simulink model "gm_NCO_32"  (R2023b)
settings: Solver=VariableStepAuto  StartTime=0.0  StopTime=100  RelTol=1e-3
undefined symbols (not defined in the file or in its folder): bhi
libraries: dsphdlfiltering2 x1, dsphdlsigops2 x1
settings Model: Creator=31651  LastModifiedBy=31651
settings OptimizationCC: BlockReduction=off  ConditionallyExecuteInputs=off  DefaultParameterBehavior=Inlined
settings DebuggingCC: AlgebraicLoopMsg=error  InheritedTsInSrcMsg=none
settings HardwareCC: ProdBitPerPointer=32  ProdBitPerSizeT=32  ProdBitPerPtrDiffT=32  ProdLargestAtomicFloat=None  ProdIntDivRoundTo=Undefined  ProdEndianess=Unspecified  ProdWordSize=32  ProdHWDeviceType=ASIC/FPGA->ASIC/FPGA  TargetBitPerPointer=64  TargetBitPerSizeT=64  TargetBitPerPtrDiffT=64  TargetLongLongMode=on  TargetIntDivRoundTo=Zero  TargetEndianess=LittleEndian  TargetWordSize=64  TargetHWDeviceType=Custom Processor->MATLAB Host Computer  ProdEqTarget=off

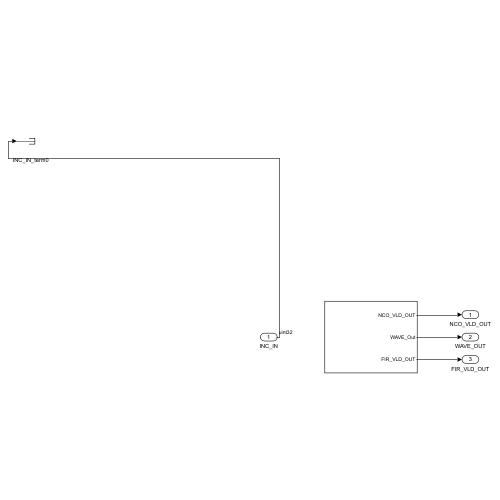
[thumbnail: Simulink's stored preview of the top-level diagram]
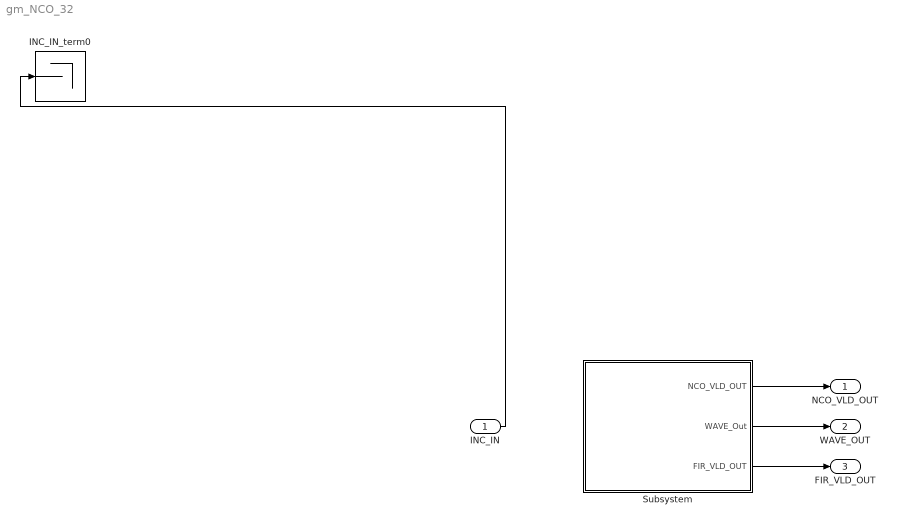
== system gm_NCO_32 ==
  INC_IN : Inport  OutDataTypeStr=uint32  PortDimensions=1  SampleTime=0.001
  INC_IN_term0 : Terminator
  Subsystem : Subsystem
  NCO_VLD_OUT : Outport  SampleTime=0.001  VectorParamsAs1DForOutWhenUnconnected=off
  WAVE_OUT : Outport  Port=2  SampleTime=0.001  VectorParamsAs1DForOutWhenUnconnected=off
  FIR_VLD_OUT : Outport  Port=3  SampleTime=0.001  VectorParamsAs1DForOutWhenUnconnected=off
  wires:
  INC_IN/1 -> INC_IN_term0/1
  Subsystem/1(NCO_VLD_OUT) -> NCO_VLD_OUT/1
  Subsystem/2(WAVE_Out) -> WAVE_OUT/1
  Subsystem/3(FIR_VLD_OUT) -> FIR_VLD_OUT/1

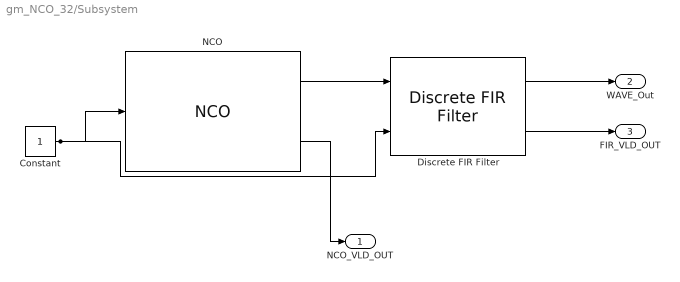
== system gm_NCO_32/Subsystem ==
  Constant : Constant  OutDataTypeStr=boolean  SampleTime=0.001
  Discrete FIR Filter : dsphdlfiltering2/Discrete FIR Filter  NumeratorSource=Property  Numerator=bhi  NumeratorPrototype=[]  FilterStructure=Direct form systolic  SerializationOption=Minimum number of cycles between valid input samples  NumCycles=2  NumberOfMultipliers=2  SimulateUsing=Code generation  roundingMode=Floor  overflowMode=off  CoefficientsDataTypeStr=Inherit: Same word length as input  OutputDataTypeStr=Inherit: Same word length as input  ResetInputPort=off  HDLGlobalReset=off  CoeffMultiplier=Multiplier  UseMultForPow2Coeff=on
  NCO : dsphdlsigops2/NCO  PhaseIncrementSource=Property  PhaseIncrement=65535  PhaseOffsetSource=Property  PhaseOffset=0  DitherSource=Property  NumDitherBits=4  SamplesPerFrame=1  LUTCompress=off  ResetAction=off  Waveform=Sine  PhasePort=off  SimulateUsing=Code generation  AccumulatorWL=16  PhaseQuantization=on  NumQuantizerAccumulatorBits=12  OutputDataType=Binary point scaling  OutputWL=16  OutputFL=14
      settings: LibrarySourceBlock=dsphdlsrcs2/NCO
  NCO_VLD_OUT : Outport  SampleTime=0.001  VectorParamsAs1DForOutWhenUnconnected=off
  WAVE_Out : Outport  Port=2  SampleTime=0.001  VectorParamsAs1DForOutWhenUnconnected=off
  FIR_VLD_OUT : Outport  Port=3  SampleTime=0.001  VectorParamsAs1DForOutWhenUnconnected=off
  wires:
  Constant/1 -> Discrete FIR Filter/2, NCO/1
  Discrete FIR Filter/1 -> WAVE_Out/1
  Discrete FIR Filter/2 -> FIR_VLD_OUT/1
  NCO/1 -> Discrete FIR Filter/1
  NCO/2 -> NCO_VLD_OUT/1
